simulink model "lab2sim"  (R2018b)
settings: Solver=FixedStepAuto  StartTime=0.0  StopTime=3.0  FixedStep=0.01  RelTol=1e-3
values from neighbouring files (symbols this model uses):
  h = 0.01    [lab2.m]
  tau = (0.031 + 0.044 + 0.097) / 3    (= 0.0573333333333)    [lab2.m]
  z1 = z(i)    [lab2.m]
settings Model: Creator=mert  LastModifiedBy=Oguz

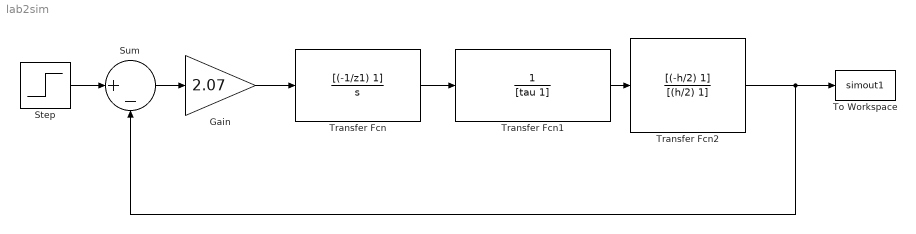
== system lab2sim ==
  Gain : Gain  Gain=2.07
  Step : Step  Time=0  After=10  SampleTime=0
  Sum : Sum  Inputs=|+-
  To Workspace : ToWorkspace  VariableName=simout1  SaveFormat=Timeseries  SampleTime=-1
  Transfer Fcn : TransferFcn  Numerator=[(-1/z1) 1]  Denominator=[1 0]
  Transfer Fcn1 : TransferFcn  Denominator=[tau 1]
  Transfer Fcn2 : TransferFcn  Numerator=[(-h/2) 1]  Denominator=[(h/2) 1]
  wires:
  Gain/1 -> Transfer Fcn/1
  Sum/1 -> Gain/1
  Transfer Fcn1/1 -> Transfer Fcn2/1
  Step/1 -> Sum/1
  Transfer Fcn/1 -> Transfer Fcn1/1
  Transfer Fcn2/1 -> To Workspace/1, Sum/2
